simulink model "Main"  (R2019a)
settings: Solver=VariableStepAuto  StartTime=0.0  StopTime=2  RelTol=1e-3
libraries: powerlib x25, eeTransforms x3, powerlib_meascontrol x3, dsparch4 x1, eeHysteresisControl x1
settings Model: Creator=Venkat koushik  LastModifiedBy=Venkat koushik
settings DataIOCC: ReturnWorkspaceOutputs=off

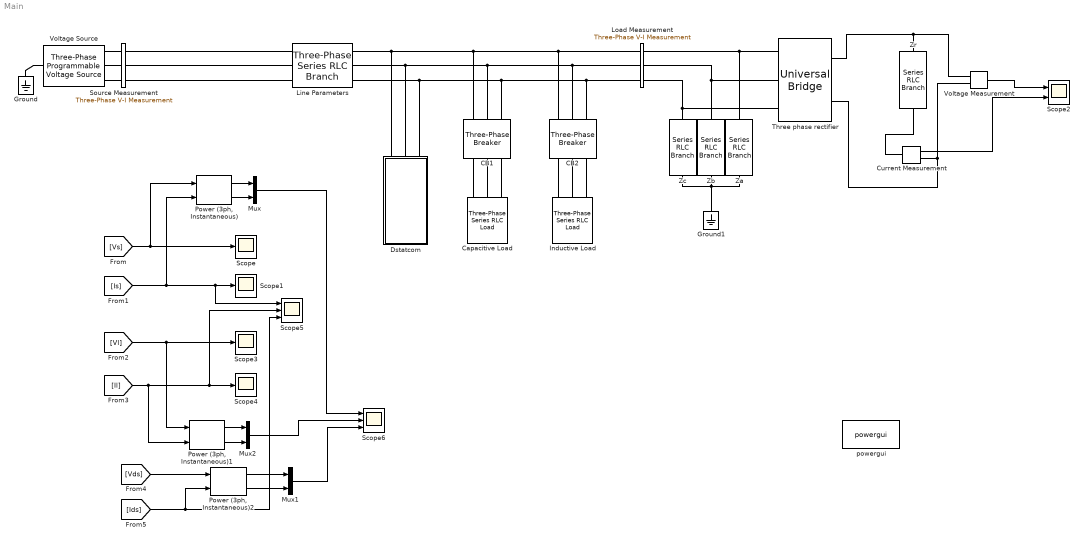
== system Main ==
  CB1 : powerlib/Elements/Three-Phase Breaker  InitialState=open  SwitchA=on  SwitchB=on  SwitchC=on  SwitchTimes=0.2  External=off  BreakerResistance=0.01  SnubberResistance=1e6  SnubberCapacitance=inf  Measurements=None
      settings: SourceProductName=Simscape Electrical
  "CB2 " : powerlib/Elements/Three-Phase Breaker  InitialState=open  SwitchA=on  SwitchB=on  SwitchC=on  SwitchTimes=0.1  External=off  BreakerResistance=0.01  SnubberResistance=1e6  SnubberCapacitance=inf  Measurements=None
      settings: SourceProductName=Simscape Electrical
  Capacitive Load : powerlib/Elements/Three-Phase Series RLC Load  LConnTagsString=A|B|C  Configuration=Y (grounded)  NominalVoltage=200  Vabc=[1e3 1e3 1e3]  Vabcp=[1e3 1e3 1e3]  NominalFrequency=50  UnbalancedPower=off  ActivePower=1000  InductivePower=0  CapacitivePower=2000  Pabc=[10e3 9e3 11e3]  QLabc=[100 90 110]  QCabc=[100 90 110]  Pabcp=[10e3 9e3 11e3]  QLabcp=[100 90 110]  QCabcp=[100 90 110]  Measurements=None  LoadType=constant Z
      settings: SourceProductName=Simscape Electrical
  Current Measurement : powerlib/Measurements/Current Measurement  PhasorSimulation=off  OutputType=Complex  PSBequivalent=0
      settings: SourceProductName=Simscape Electrical
  Dstatcom : Subsystem
  Ground : powerlib/Elements/Ground  LConnTagsString=a
      settings: SourceProductName=Simscape Electrical
  Ground1 : powerlib/Elements/Ground  LConnTagsString=a
      settings: SourceProductName=Simscape Electrical
  Inductive Load : powerlib/Elements/Three-Phase Series RLC Load  LConnTagsString=A|B|C  Configuration=Y (grounded)  NominalVoltage=200  Vabc=[1e3 1e3 1e3]  Vabcp=[1e3 1e3 1e3]  NominalFrequency=50  UnbalancedPower=off  ActivePower=1000  InductivePower=1000  CapacitivePower=0  Pabc=[10e3 9e3 11e3]  QLabc=[100 90 110]  QCabc=[100 90 110]  Pabcp=[10e3 9e3 11e3]  QLabcp=[100 90 110]  QCabcp=[100 90 110]  Measurements=None  LoadType=constant Z
      settings: SourceProductName=Simscape Electrical
  Line Parameters : powerlib/Elements/Three-Phase Series RLC Branch  LConnTagsString=A|B|C  RConnTagsString=A|B|C  BranchType=RL  Resistance=1  Inductance=0.1e-3  Capacitance=1e-6  Measurements=None
      settings: SourceProductName=Simscape Electrical
  Load Measurement : powerlib/Measurements/Three-Phase V-I Measurement  VoltageMeasurement=phase-to-ground  SetLabelV=on  LabelV=Vl  Vpu=off  VpuLL=off  CurrentMeasurement=yes  SetLabelI=on  LabelI=Il  Ipu=off  Pbase=100e6  Vbase=500e3  OutputType=Complex  PhasorSimulation=off  PSBequivalent=0
      settings: SourceProductName=Simscape Electrical
  Mux : Mux  Inputs=2
  Mux1 : Mux  Inputs=2
  Mux2 : Mux  Inputs=2
  "Power (3ph, Instantaneous)" : powerlib_meascontrol/Measurements/Power (3ph, Instantaneous)
      settings: SourceProductName=Simscape Electrical
  "Power (3ph, Instantaneous)1" : powerlib_meascontrol/Measurements/Power (3ph, Instantaneous)
      settings: SourceProductName=Simscape Electrical
  "Power (3ph, Instantaneous)2" : powerlib_meascontrol/Measurements/Power (3ph, Instantaneous)
      settings: SourceProductName=Simscape Electrical
  Scope{,1,3..4} (4 alike) : Scope
  Scope2 : Scope  NumInputPorts=2
  Scope5 : Scope  NumInputPorts=3
  Scope6 : Scope  NumInputPorts=3
  Source Measurement : powerlib/Measurements/Three-Phase V-I Measurement  VoltageMeasurement=phase-to-ground  SetLabelV=on  LabelV=Vs  Vpu=off  VpuLL=off  CurrentMeasurement=yes  SetLabelI=on  LabelI=Is  Ipu=off  Pbase=100e6  Vbase=500e3  OutputType=Complex  PhasorSimulation=off  PSBequivalent=0
      settings: SourceProductName=Simscape Electrical
  Three phase rectifier : powerlib/Power Electronics/Universal Bridge  Arms=3  SnubberResistance=1e5  SnubberCapacitance=inf  Device=Diodes  Ron=1e-3  Lon=0  ForwardVoltages="[  0  0  ]"  ForwardVoltage=0  GTOparameters=[ 10e-6 , 20e-6 ]  IGBTparameters=[ 1e-6 , 2e-6 ]  Measurements=None  Measurements_2=None  converterType=Rectifier
      settings: SourceProductName=Simscape Electrical
  Voltage Measurement : powerlib/Measurements/Voltage Measurement  PhasorSimulation=off  OutputType=Complex  PSBequivalent=0
      settings: SourceProductName=Simscape Electrical
  Voltage Source : powerlib/Electrical Sources/Three-Phase Programmable Voltage Source  PositiveSequence=[200 0 50]  VariationEntity=None  VariationType=Table of time-amplitude pairs  VariationTypeAlt=Step  VariationStep=0.5  VariationRate=10  VariationMagnitude=0.3  VariationFrequency=2  VariationTiming=[1 2]  VariationPhaseA=off  Amplitudes=[1 0.8 1.2 1.0]  TimeValues=[0 0.1 0.15 0.2]  HarmonicGeneration=off  HarmonicA=[3 0.2 -25 0]  HarmonicB=[2 0.15 35 2]  Timing="[0.05  3]"  BusType=swing  Pref=0  Qref=0  Qmin=-inf  Qmax=inf
      settings: SourceProductName=Simscape Electrical
  Za : powerlib/Elements/Series RLC Branch  LConnTagsString=__new0  RConnTagsString=__new0  BranchType=RL  Resistance=200  Inductance=103/(2*pi*50)  SetiL0=off  InitialCurrent=0  Capacitance=1e-6  Setx0=off  InitialVoltage=0  Measurements=None
      settings: SourceProductName=Simscape Electrical
  Zb : powerlib/Elements/Series RLC Branch  LConnTagsString=__new0  RConnTagsString=__new0  BranchType=RL  Resistance=160  Inductance=63/(2*pi*50)  SetiL0=off  InitialCurrent=0  Capacitance=1e-6  Setx0=off  InitialVoltage=0  Measurements=None
      settings: SourceProductName=Simscape Electrical
  Zc : powerlib/Elements/Series RLC Branch  LConnTagsString=__new0  RConnTagsString=__new0  BranchType=RL  Resistance=100  Inductance=110/(2*pi*50)  SetiL0=off  InitialCurrent=0  Capacitance=1e-6  Setx0=off  InitialVoltage=0  Measurements=None
      settings: SourceProductName=Simscape Electrical
  Zr : powerlib/Elements/Series RLC Branch  LConnTagsString=__new0  RConnTagsString=__new0  BranchType=RL  Resistance=120  Inductance=63/(2*pi*50)  SetiL0=off  InitialCurrent=0  Capacitance=1e-6  Setx0=off  InitialVoltage=0  Measurements=None
      settings: SourceProductName=Simscape Electrical
  powergui : powerlib/powergui  Priority=1  SimulationMode=Discrete  SampleTime=5e-6  frequency=60  Iterations=50  frequencyindice=0  Pbase=100e6  ErrMax=1e-4  UnitsV=kV  UnitsW=MW  buscounter=0  FunctionMessages=off  echomessages=off  EnableUseOfTLC=off  CurrentSourceSwitches=off  DisableSnubberDevices=off  DisableRonSwitches=off  DisableVfSwitches=off  DisplayEquations=off  AutomaticDiscreteSolvers=off  SolverType=Tustin/Backward Euler (TBE)  Interpol=off  ExternalGateDelay=off  methode=off  Ts=100  x0status=blocks  SPID=on  SwTol=0  HookPort=off  NonlinearTolerance=0  nMaxIteration=15  ContinueOnMaxIteration=off  RestoreLinks=warning  ResistiveCurrentMeasurement=off  Frange=[0:2:500]  Ylog=off  Xlog=on  ShowGrid=off  save=off  variable=ZData  structure=Sourcecurrent  ZoomFFT=off  StartTime=.25  cycles=1  DisplayStyle=1  fundamental=50  FreqAxis=off  MaxFrequency=1000  frequencyindicesteady=1  RmsSteady=1  display=off
      settings: SourceProductName=Simscape Electrical
  wires:
  Voltage Measurement/1 -> Scope2/1
  Current Measurement/1 -> Scope2/2
  [Vs] -> "Power (3ph, Instantaneous)"/1, Scope/1
  [Is] -> "Power (3ph, Instantaneous)"/2, Scope5/1, Scope1/1
  [Vl] -> "Power (3ph, Instantaneous)1"/1, Scope3/1
  [Il] -> "Power (3ph, Instantaneous)1"/2, Scope5/2, Scope4/1
  [Ids] -> "Power (3ph, Instantaneous)2"/2, Scope5/3
  [Vds] -> "Power (3ph, Instantaneous)2"/1
  "Power (3ph, Instantaneous)"/1 -> Mux/1
  "Power (3ph, Instantaneous)"/2 -> Mux/2
  "Power (3ph, Instantaneous)2"/1 -> Mux1/1
  "Power (3ph, Instantaneous)2"/2 -> Mux1/2
  "Power (3ph, Instantaneous)1"/1 -> Mux2/1
  "Power (3ph, Instantaneous)1"/2 -> Mux2/2
  Mux/1 -> Scope6/1
  Mux2/1 -> Scope6/2
  Mux1/1 -> Scope6/3
  connections:
  Voltage Source/LConn1 -- Ground/LConn1
  Source Measurement/LConn1 -- Voltage Source/RConn1
  Source Measurement/LConn2 -- Voltage Source/RConn2
  Source Measurement/LConn3 -- Voltage Source/RConn3
  Source Measurement/RConn2 -- Line Parameters/LConn2
  Line Parameters/LConn1 -- Source Measurement/RConn1
  Line Parameters/LConn3 -- Source Measurement/RConn3
  Load Measurement/LConn1 -- Line Parameters/RConn1 -- Dstatcom/LConn1 -- CB1/RConn1 -- "CB2 "/RConn1
  Three phase rectifier/LConn1 -- Load Measurement/RConn1 -- Za/RConn1
  Three phase rectifier/LConn2 -- Zb/RConn1 -- Load Measurement/RConn2
  Three phase rectifier/LConn3 -- Zc/RConn1 -- Load Measurement/RConn3
  Ground1/LConn1 -- Zc/LConn1 -- Za/LConn1 -- Zb/LConn1
  Zr/LConn1 -- Voltage Measurement/LConn1 -- Three phase rectifier/RConn1
  Current Measurement/RConn1 -- Voltage Measurement/LConn2 -- Three phase rectifier/RConn2
  Current Measurement/LConn1 -- Zr/RConn1
  Load Measurement/LConn2 -- Dstatcom/LConn2 -- Line Parameters/RConn2 -- CB1/RConn2 -- "CB2 "/RConn2
  Load Measurement/LConn3 -- "CB2 "/RConn3 -- CB1/RConn3 -- Dstatcom/LConn3 -- Line Parameters/RConn3
  Capacitive Load/LConn3 -- CB1/LConn3
  CB1/LConn2 -- Capacitive Load/LConn2
  CB1/LConn1 -- Capacitive Load/LConn1
  "CB2 "/LConn1 -- Inductive Load/LConn1
  Inductive Load/LConn2 -- "CB2 "/LConn2
  Inductive Load/LConn3 -- "CB2 "/LConn3

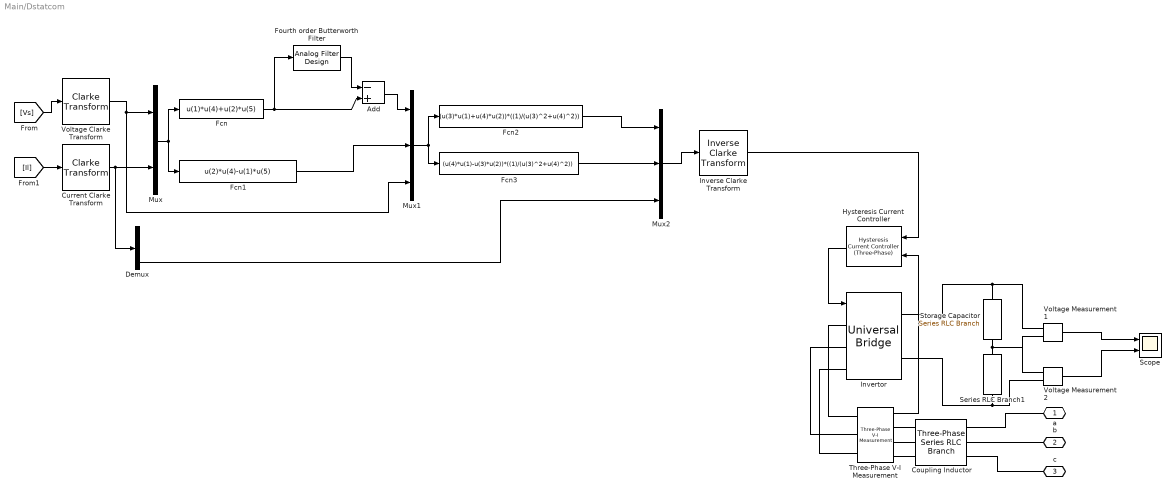
== system Main/Dstatcom ==
  Add : Sum  Inputs=-+
  "Coupling Inductor " : powerlib/Elements/Three-Phase Series RLC Branch  LConnTagsString=A|B|C  RConnTagsString=A|B|C  BranchType=L  Resistance=1  Inductance=7e-3  Capacitance=1e-6  Measurements=None
      settings: SourceProductName=Simscape Electrical
  Current Clarke Transform : eeTransforms/Clarke Transform  PowerInvariant=off
      settings: SourceProductName=Simscape Electrical  SourceProductBaseCode=PS
  Demux : Demux  Outputs=3
  Fcn : Fcn  Expr=u(1)*u(4)+u(2)*u(5)
  Fcn1 : Fcn  Expr=u(2)*u(4)-u(1)*u(5)
  Fcn2 : Fcn  Expr=(u(3)*u(1)+u(4)*u(2))*((1)/(u(3)^2+u(4)^2))
  Fcn3 : Fcn  Expr=(u(4)*u(1)-u(3)*u(2))*((1)/(u(3)^2+u(4)^2))
  Fourth order Butterworth Filter : dsparch4/Analog Filter Design  method=Butterworth  filttype=Lowpass  N=4  Wlo=2*pi*50  Whi=80  Rp=2  Rs=40
  "Hysteresis Current Controller " : eeHysteresisControl/Hysteresis Current Controller (Three-Phase)  h=0.02  Ts=-1
      settings: SourceProductName=Simscape Electrical  SourceProductBaseCode=PS
  Inverse Clarke Transform : eeTransforms/Inverse Clarke Transform  PowerInvariant=off
      settings: SourceProductName=Simscape Electrical  SourceProductBaseCode=PS
  Invertor : powerlib/Power Electronics/Universal Bridge  Arms=3  SnubberResistance=1e5  SnubberCapacitance=inf  Device=IGBT / Diodes  Ron=1e-3  Lon=0  ForwardVoltages="[  0  0  ]"  ForwardVoltage=0  GTOparameters=[ 10e-6 , 20e-6 ]  IGBTparameters=[ 1e-6 , 2e-6 ]  Measurements=None  Measurements_2=None  converterType=Rectifier
      settings: SourceProductName=Simscape Electrical
  Mux : Mux  Inputs=2
  Mux1 : Mux  Inputs=3
  Mux2 : Mux  Inputs=3
  Scope : Scope  NumInputPorts=2
  Series RLC Branch1 : powerlib/Elements/Series RLC Branch  LConnTagsString=__new0  RConnTagsString=__new0  BranchType=C  Resistance=1  Inductance=1e-3  SetiL0=off  InitialCurrent=0  Capacitance=600e-6  Setx0=off  InitialVoltage=0  Measurements=None
      settings: SourceProductName=Simscape Electrical
  Storage Capacitor : powerlib/Elements/Series RLC Branch  LConnTagsString=__new0  RConnTagsString=__new0  BranchType=C  Resistance=1  Inductance=1e-3  SetiL0=off  InitialCurrent=0  Capacitance=600e-9  Setx0=off  InitialVoltage=0  Measurements=None
      settings: SourceProductName=Simscape Electrical
  Three-Phase V-I Measurement : powerlib/Measurements/Three-Phase V-I Measurement  VoltageMeasurement=phase-to-ground  SetLabelV=on  LabelV=Vabc  Vpu=off  VpuLL=off  CurrentMeasurement=yes  SetLabelI=off  LabelI=Iabc  Ipu=off  Pbase=100e6  Vbase=500e3  OutputType=Complex  PhasorSimulation=off  PSBequivalent=0
      settings: SourceProductName=Simscape Electrical
  Voltage Clarke Transform : eeTransforms/Clarke Transform  PowerInvariant=off
      settings: SourceProductName=Simscape Electrical  SourceProductBaseCode=PS
  Voltage Measurement1 : powerlib/Measurements/Voltage Measurement  PhasorSimulation=off  OutputType=Complex  PSBequivalent=0
      settings: SourceProductName=Simscape Electrical
  Voltage Measurement2 : powerlib/Measurements/Voltage Measurement  PhasorSimulation=off  OutputType=Complex  PSBequivalent=0
      settings: SourceProductName=Simscape Electrical
  a : PMIOPort  Side=Left
  b : PMIOPort  Port=2  Side=Left
  c : PMIOPort  Port=3  Side=Left
  wires:
  [Vs] -> Voltage Clarke Transform/1
  Voltage Clarke Transform/1 -> Mux1/3, Mux/1
  [Il] -> Current Clarke Transform/1
  Current Clarke Transform/1 -> Demux/1, Mux/2
  Mux/1 -> Fcn1/1, Fcn/1
  Fcn/1 -> Add/2, Fourth order Butterworth Filter/1
  Fourth order Butterworth Filter/1 -> Add/1
  Fcn1/1 -> Mux1/2
  Add/1 -> Mux1/1
  Mux1/1 -> Fcn3/1, Fcn2/1
  Demux/3 -> Mux2/3
  Fcn3/1 -> Mux2/2
  Fcn2/1 -> Mux2/1
  Mux2/1 -> Inverse Clarke Transform/1
  Inverse Clarke Transform/1 -> "Hysteresis Current Controller "/1
  Three-Phase V-I Measurement/1 -> "Hysteresis Current Controller "/2
  Voltage Measurement1/1 -> Scope/1
  Voltage Measurement2/1 -> Scope/2
  "Hysteresis Current Controller "/1 -> Invertor/1
  connections:
  Invertor/RConn1 -- Voltage Measurement1/LConn1 -- Storage Capacitor/LConn1
  Series RLC Branch1/LConn1 -- Voltage Measurement2/LConn1 -- Voltage Measurement1/LConn2 -- Storage Capacitor/RConn1
  Invertor/RConn2 -- Voltage Measurement2/LConn2 -- Series RLC Branch1/RConn1
  Three-Phase V-I Measurement/LConn1 -- Invertor/LConn1
  Three-Phase V-I Measurement/LConn2 -- Invertor/LConn2
  Invertor/LConn3 -- Three-Phase V-I Measurement/LConn3
  "Coupling Inductor "/LConn1 -- Three-Phase V-I Measurement/RConn1
  "Coupling Inductor "/LConn2 -- Three-Phase V-I Measurement/RConn2
  Three-Phase V-I Measurement/RConn3 -- "Coupling Inductor "/LConn3
  "Coupling Inductor "/RConn1 -- a/RConn1
  b/RConn1 -- "Coupling Inductor "/RConn2
  c/RConn1 -- "Coupling Inductor "/RConn3
